simulink model "A1a"  (R2025b)
settings: Solver=FixedStepAuto  StartTime=0.0  StopTime=20  FixedStep=0.001  RelTol=1e-3
values from neighbouring files (symbols this model uses):
  k1 = (m*l)/(m*l^2+J)    (= 1.25)    [Lab1.m]
  k2 = (m*g*l)/(m*l^2+J)    (= 12.2625)    [Lab1.m]
  k3 = (c_r)/(m*l^2+J)    (= 0.3125)    [Lab1.m]
settings Model: Creator=david  LastModifiedBy=david

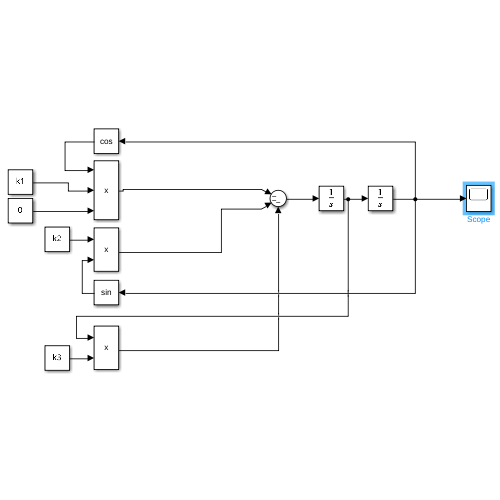
[thumbnail: Simulink's stored preview of the top-level diagram]
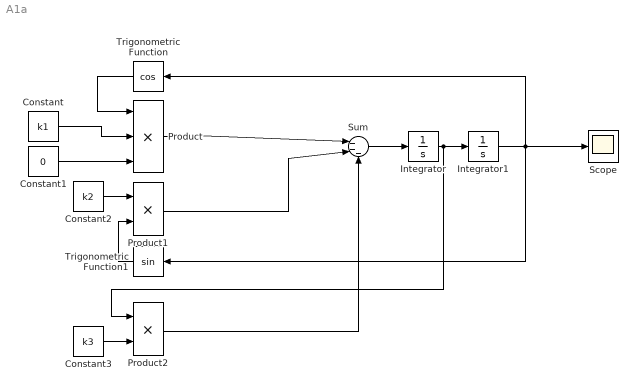
== system A1a ==
  Constant : Constant  Value=k1
  Constant1 : Constant  Value=0
  Constant2 : Constant  Value=k2
  Constant3 : Constant  Value=k3
  Integrator : Integrator
  Integrator1 : Integrator  InitialCondition=pi/2
  Product : Product  Inputs=3
  Product1 : Product
  Product2 : Product
  Scope : Scope
      settings: ActiveDisplayYMinimum=-2.8843235461268657  ActiveDisplayYMaximum=3.5121066434972583
  Sum : Sum  Inputs=|---
  Trigonometric Function : Trigonometry  Operator=cos
  Trigonometric Function1 : Trigonometry
  wires:
  Integrator/1 -> Product2/1, Integrator1/1
  Integrator1/1 -> Trigonometric Function/1, Scope/1, Trigonometric Function1/1
  Constant/1 -> Product/2
  Constant1/1 -> Product/3
  Trigonometric Function/1 -> Product/1
  Product/1 -> Sum/1
  Constant2/1 -> Product1/1
  Trigonometric Function1/1 -> Product1/2
  Product1/1 -> Sum/2
  Product2/1 -> Sum/3
  Constant3/1 -> Product2/2
  Sum/1 -> Integrator/1
